simulink subsystem "EcDiferenciales"  (R2023b)
settings: Solver=VariableStepAuto  StartTime=0.0  StopTime=10.0  RelTol=1e-3
libraries: arduinosensorlib x2
settings Model: Creator=Hajar  LastModifiedBy=Hajar

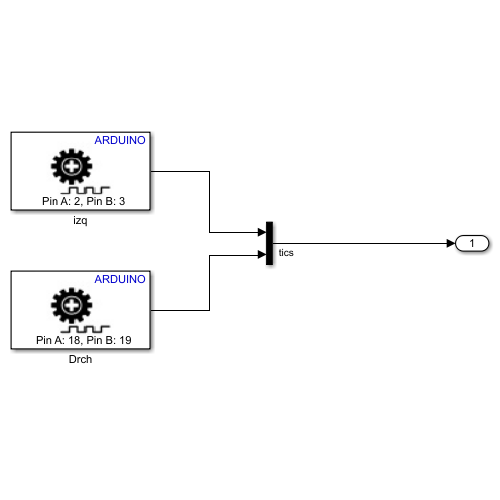
[thumbnail: Simulink's stored preview of the top-level diagram]
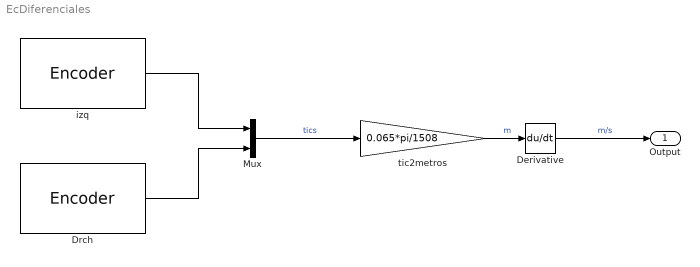
== system EcDiferenciales ==
  Derivative : Derivative
  Drch : arduinosensorlib/Encoder  InputA=18  InputB=19  Mode=No reset  SampleTime=-1
  Mux : Mux  Inputs=2
  izq : arduinosensorlib/Encoder  InputA=2  InputB=3  Mode=No reset  SampleTime=-1
  tic2metros : Gain  Gain=0.065*pi/1508  OutDataTypeStr=double
  Output : Outport
  wires:
  izq/1 -> Mux/1
  Drch/1 -> Mux/2
  Mux/1 -> tic2metros/1  "tics"
  tic2metros/1 -> Derivative/1  "m"
  Derivative/1 -> Output/1  "m/s"
